simulink model "ZeroDoF"  (R2024a)
settings: Solver=VariableStepAuto  StartTime=0.0  StopTime=10  RelTol=1e-3
undefined symbols (not defined in the file): Cd, g, m, rho
settings Model: Creator=samuj  LastModifiedBy=samuj

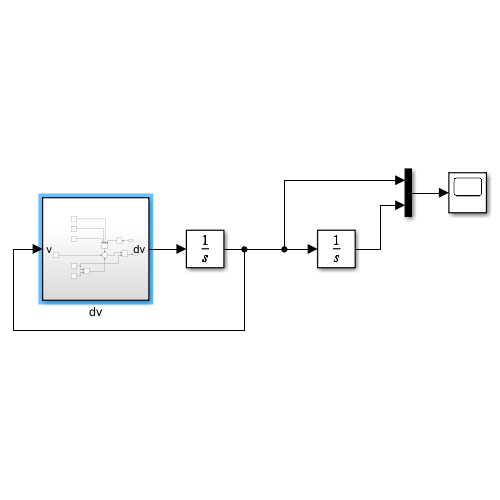
[thumbnail: Simulink's stored preview of the top-level diagram]
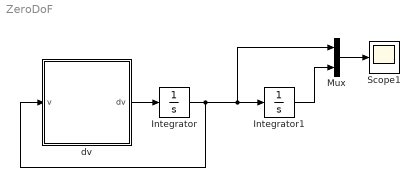
== system ZeroDoF ==
  Integrator : Integrator
  Integrator1 : Integrator
  Mux : Mux  Inputs=2
  Scope1 : Scope
  dv : Subsystem
  wires:
  Integrator/1 -> dv/1(v), Mux/1, Integrator1/1
  Mux/1 -> Scope1/1
  Integrator1/1 -> Mux/2
  dv/1(dv) -> Integrator/1

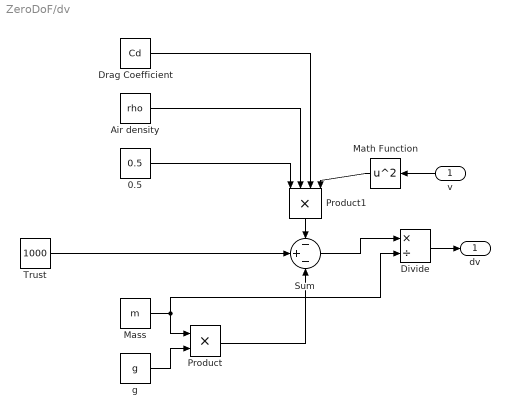
== system ZeroDoF/dv ==
  v : Inport
  0.5 : Constant  Value=0.5
  Air density : Constant  Value=rho
  Divide : Product  Inputs=*/
  Drag Coefficient : Constant  Value=Cd
  Mass : Constant  Value=m
  Math Function : Math  Operator=square
  Product : Product
  Product1 : Product  Inputs=4
  Sum : Sum  Inputs=-+-
  Trust : Constant  Value=1000
  g : Constant  Value=g
  dv : Outport
  wires:
  v/1 -> Math Function/1
  0.5/1 -> Product1/1
  Product1/1 -> Sum/1
  g/1 -> Product/2
  Mass/1 -> Divide/2, Product/1
  Drag Coefficient/1 -> Product1/3
  Math Function/1 -> Product1/4
  Product/1 -> Sum/3
  Trust/1 -> Sum/2
  Air density/1 -> Product1/2
  Sum/1 -> Divide/1
  Divide/1 -> dv/1
